simulink subsystem "discrete_reduced_order_observer"  (R2024b)
settings: Solver=VariableStepAuto  StartTime=0.0  StopTime=10.0  RelTol=1e-3
values from neighbouring files (symbols this model uses):
  Ts = Ts_values(i)    [A_final_results.m]
settings Model: Creator=Riccardo Grosso  LastModifiedBy=Buton

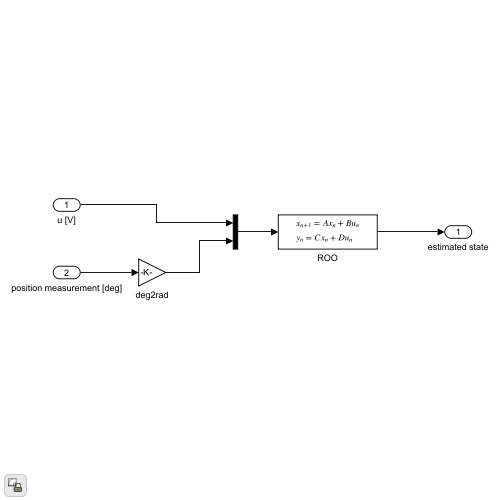
[thumbnail: Simulink's stored preview of the top-level diagram]
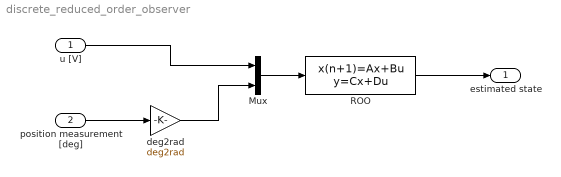
== system discrete_reduced_order_observer ==
  u [V] : Inport
  position measurement [deg] : Inport  Port=2
  Mux : Mux  Inputs=2
  ROO : DiscreteStateSpace  A=0.000212192189233434  B=[3.2485889488403 -7.73934237483777]  C=[0;1]  D=[0 1;0 7.74098495138143]  SampleTime=Ts
  deg2rad : Gain  Gain=deg2rad
  estimated state : Outport
  wires:
  position measurement [deg]/1 -> deg2rad/1
  Mux/1 -> ROO/1
  u [V]/1 -> Mux/1
  deg2rad/1 -> Mux/2
  ROO/1 -> estimated state/1
